simulink model "Flightgear_Tester"  (Simulink 7.8)
settings: Solver=FixedStepDiscrete  SolverMode=SingleTasking  StartTime=0.0  StopTime=inf  FixedStep=dt_sim  RelTol=1e-3
values from neighbouring files (symbols this model uses):
  D = 1    [Init.m]
  dt_sim = 0.005    [Init.m]
undefined symbols (not defined in the file or in its folder): scenario, vis, waitfortreal
settings Model: Creator=ft14sl  LastModifiedBy=ft14sl
settings DataIOCC: LimitDataPoints=off  SaveOutput=off  SignalLogging=off  DSMLogging=off  SaveTime=off
settings DebuggingCC: ConsistencyChecking=error  SignalInfNanChecking=error  SignalRangeChecking=error  AlgebraicLoopMsg=error  ArtificialAlgebraicLoopMsg=error  SaveWithDisabledLinksMsg=error  SaveWithParameterizedLinksMsg=error  UnderspecifiedInitializationDetection=Simplified  MergeDetectMultiDrivingBlocksExec=error  BlockPriorityViolationMsg=error  MinStepSizeMsg=error  TimeAdjustmentMsg=warning  SolverPrmCheckMsg=error  InheritedTsInSrcMsg=error  DiscreteInheritContinuousMsg=error  SingleTaskRateTransMsg=error  TasksWithSamePriorityMsg=error  SigSpecEnsureSampleTimeMsg=error  CheckMatrixSingularityMsg=error  IntegerOverflowMsg=error  ParameterUnderflowMsg=error  ParameterPrecisionLossMsg=error  ParameterTunabilityLossMsg=error  FixptConstUnderflowMsg=error  FixptConstOverflowMsg=error  FixptConstPrecisionLossMsg=error  UnderSpecifiedDataTypeMsg=error  UnnecessaryDatatypeConvMsg=warning  VectorMatrixConversionMsg=error  SignalLabelMismatchMsg=error  UnconnectedInputMsg=error  UnconnectedOutputMsg=error  UnconnectedLineMsg=error  SFcnCompatibilityMsg=error  UniqueDataStoreMsg=error  BusObjectLabelMismatch=error  RootOutportRequireBusObject=error  ModelReferenceIOMsg=error  ModelReferenceVersionMismatchMessage=error  ModelReferenceIOMismatchMessage=error  ModelReferenceCSMismatchMessage=error  UnknownTsInhSupMsg=error  ModelReferenceDataLoggingMessage=error  SimStateInterfaceChecksumMismatchMsg=error  StrictBusMsg=ErrorOnBusTreatedAsVector  NonBusSignalsTreatedAsBus=error  SFUnusedDataAndEventsDiag=error  SFUnexpectedBacktrackingDiag=error  SFInvalidInputDataAccessInChartInitDiag=error  SFNoUnconditionalDefaultTransitionDiag=error  SFTransitionOutsideNaturalParentDiag=error  SFUnconditionalTransitionShadowingDiag=error

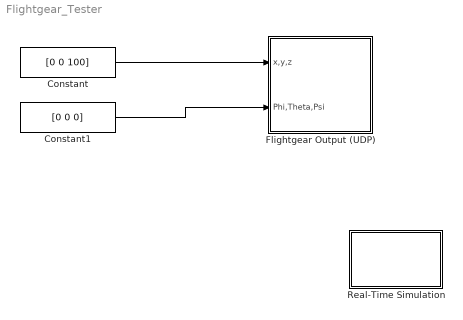
== system Flightgear_Tester ==
  Constant : Constant  Value=[0 0 100]
  Constant1 : Constant  Value=[0 0 0]
  Flightgear Output (UDP) : Subsystem  TreatAsAtomicUnit=on
  Real-Time Simulation : Subsystem
      mask Display: disp('SL RT')
  wires:
  Constant/1 -> Flightgear Output (UDP)/1(x,y,z)
  Constant1/1 -> Flightgear Output (UDP)/2(Phi,Theta,Psi)

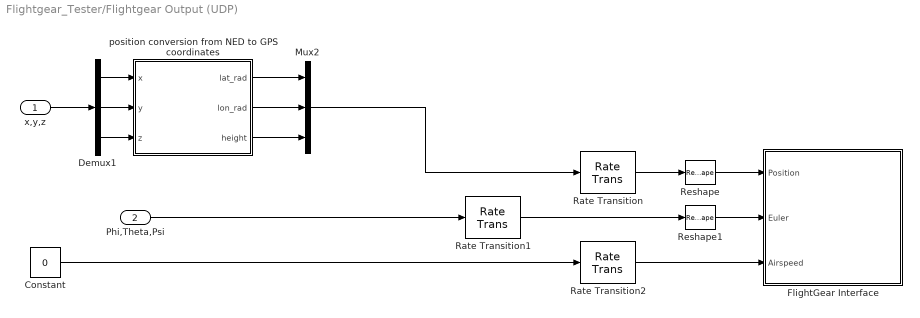
== system Flightgear_Tester/Flightgear Output (UDP) ==
  x,y,z : Inport
  Phi,Theta,Psi : Inport  Port=2
  Constant : Constant  Value=0
  Demux1 : Demux  Outputs=3
  FlightGear Interface : Subsystem  mask(FlightGear interface){hostname=vis.IP_fg, port=vis.PORT_fg, tsamp=vis.dt_vis}
      mask prompts: hostname "Host name:"; tsamp "Sample time:"
      mask help: FlightGear Flight Simulator Interface that provides a visual output of the aircraft position and attitude.
      mask Help:
      | The block provides position and attitude information to FlightGear Flight Simulator for visual output of the aircraft behavior.
      | <P><B>Parameters:</B>
      | <LI>Sample time: the sample time at which data is sent to FlightGear;</LI>
      | <LI>Host name: the name or IP address of the machine on which FlightGear is running.</LI></P>
      | <P><B>Inputs:</B>
      | <LI> the 3x1 vector of geographic position;</LI>
      | <LI> the 3x1 vector of Euler angles;</LI>
      | <LI> scalar number representing airspeed.</LI></P>
  Mux2 : Mux  Inputs=3
  Rate Transition : RateTransition
  Rate Transition1 : RateTransition
  Rate Transition2 : RateTransition
  Reshape : Reshape  OutputDimensionality=Column vector (2-D)
  Reshape1 : Reshape  OutputDimensionality=Column vector (2-D)
  position conversion from NED to GPS coordinates : Subsystem  mask{dRefLat=scenario.dRefLat, dRefLon=scenario.dRefLon, dRefAlt=scenario.dRefAlt, dt_sim=dt_sim}
      mask prompts: dRefLat "Reference Latitude (dRefLat) in rad"; dRefLon "Reference Longitude (dRefLon) in rad"; dRefAlt "Reference altitude (dRefAlt)  in rad"; dt_sim "Sample Time"
      mask init:
      | %WGS-84 semimajor axis_m
      | C_WGS84_a = 6378137.0;
      | %WGS-84 numerical eccentricity
      | C_WGS84_ECC_2=0.006694379992;
      | 
      | %small error
      | sqsinphi = (sin(dRefLat))*(sin(dRefLat)); %Phi, lateral
      | 
      | Rn = C_WGS84_a * ( 1.0 - C_WGS84_ECC_2 ) * (1.0 - C_WGS84_ECC_2*sqsinphi )^(-1.5);
      | Re = C_WGS84_a / sqrt( 1.0 - C_WGS84_ECC_2 * sqsinphi);
  wires:
  Rate Transition1/1 -> Reshape1/1
  Reshape1/1 -> FlightGear Interface/2(Euler)
  Reshape/1 -> FlightGear Interface/1(Position)
  Rate Transition2/1 -> FlightGear Interface/3(Airspeed)
  Rate Transition/1 -> Reshape/1
  Constant/1 -> Rate Transition2/1
  Phi,Theta,Psi/1 -> Rate Transition1/1
  x,y,z/1 -> Demux1/1
  Demux1/1 -> position conversion from NED to GPS coordinates/1(x)
  Demux1/2 -> position conversion from NED to GPS coordinates/2(y)
  Demux1/3 -> position conversion from NED to GPS coordinates/3(z)
  position conversion from NED to GPS coordinates/1(lat_rad) -> Mux2/1
  position conversion from NED to GPS coordinates/2(lon_rad) -> Mux2/2
  position conversion from NED to GPS coordinates/3(height) -> Mux2/3
  Mux2/1 -> Rate Transition/1

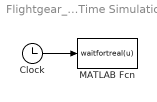
== system Flightgear_Tester/Real-Time Simulation ==
  Clock : Clock
  MATLAB Fcn : MATLABFcn  MATLABFcn=waitfortreal(u)  OutputDimensions=0
  wires:
  Clock/1 -> MATLAB Fcn/1

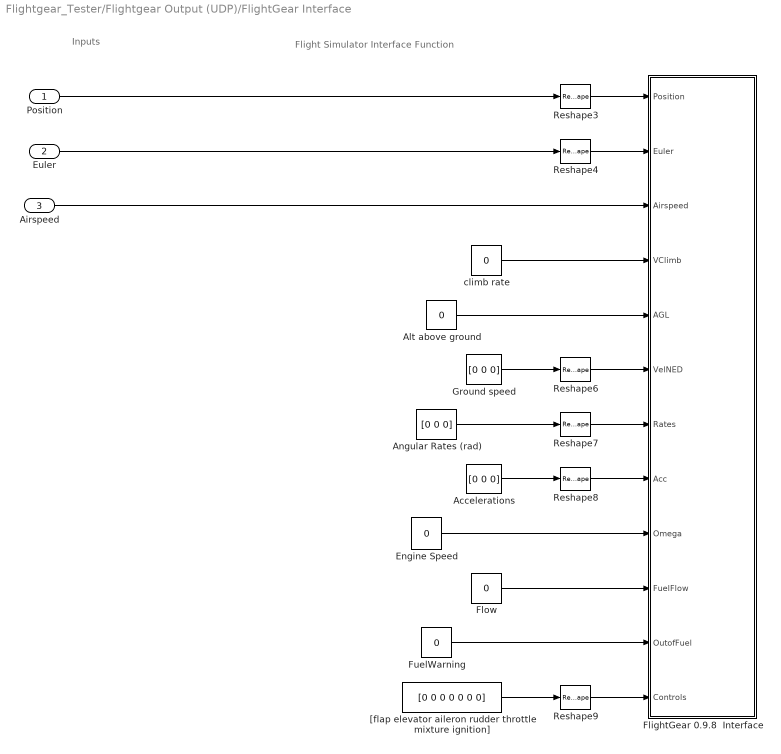
== system Flightgear_Tester/Flightgear Output (UDP)/FlightGear Interface ==
  note: Inputs
  note: Flight Simulator Interface Function
  Position : Inport  OutDataTypeStr=double  PortDimensions=[3 1]
  Euler : Inport  Port=2  OutDataTypeStr=double  PortDimensions=[3 1]
  Airspeed : Inport  Port=3  OutDataTypeStr=double  PortDimensions=1
  Accelerations : Constant  Value=[0 0 0]
  Alt above ground : Constant  Value=0
  Angular Rates (rad) : Constant  Value=[0 0 0]
  Engine Speed : Constant  Value=0
  FlightGear 0.9.8  Interface : Subsystem  mask(FlightGear 0.9.8 interface){hostname=hostname, port=port, tsamp=tsamp}
      mask prompts: hostname "Host name:"; tsamp "Sample time:"
      mask help:
      | FlightGear Flight Simulator Interface that provides a visual output of the aircraft position and attitude.
      | This driver can be used with FlightGear 0.9.8 only.
      mask Help:
      | The block provides position and attitude information to FlightGear Flight Simulator 0.9.8 for visual output of the aircraft behavior.
      | <P><B>Parameters:</B>
      | <LI>Sample time: the sample time at which data is sent to FlightGear;</LI>
      | <LI>Host name: the name or IP address of the machine on which FlightGear is running.</LI>
      | <LI>Port: the port number on the host machine.</LI>
      | </P>
      | <P><B>Inputs:</B>
      | <LI>Position =  the 3x1 vector of geographic position in [rad rad m];</LI>
      | <LI>Euler =  the 3x1 vector of Euler angles in radians;</LI>
      | <LI>Airspeed =  scalar number representing airspeed, in m/s;</LI>
      | <LI>VClimb = the climb rate, in m/s;</LI>
      | <LI>AGL = the altitude above ground, in meters;</LI>
      | <LI>VelNED = the 3x1 vector of groundspeed, in m/s;</LI>
      | <LI>Rates = the 3x1 vector of angular rates, in rad/s;</LI>
      | <LI>Acc = the 3x1 vector of body accelerations, in m/s^2;</LI>
      | <LI>Omega = the engine speed,in rad/s;</LI>
      | <LI>FuelFlow = the instananeous fuel flow, in grams per hour;</LI>
      | <LI>OutofFuel = set it to 1 to disable engine noise in FlightGear, otherwise set it to 0;</LI>
      | <LI>Controls = the 7x1 vector of aircraft controls [flap elevator aileron rudder throttle mixture ignition]; the first 4 aerodynamic controls should be normalized to [-1, 1].</LI>
      | </P>
  Flow : Constant  Value=0
  FuelWarning : Constant  Value=0
  Ground speed : Constant  Value=[0 0 0]
  Reshape{3..4,6..9} (6 alike) : Reshape  OutputDimensionality=Column vector (2-D)
  "[flap elevator aileron rudder throttle mixture ignition]" : Constant  Value=[0 0 0 0 0 0 0]
  climb rate : Constant  Value=0
  wires:
  Reshape9/1 -> FlightGear 0.9.8  Interface/12(Controls)
  Reshape8/1 -> FlightGear 0.9.8  Interface/8(Acc)
  Reshape7/1 -> FlightGear 0.9.8  Interface/7(Rates)
  Reshape6/1 -> FlightGear 0.9.8  Interface/6(VelNED)
  Reshape4/1 -> FlightGear 0.9.8  Interface/2(Euler)
  Reshape3/1 -> FlightGear 0.9.8  Interface/1(Position)
  "[flap elevator aileron rudder throttle mixture ignition]"/1 -> Reshape9/1
  FuelWarning/1 -> FlightGear 0.9.8  Interface/11(OutofFuel)
  Flow/1 -> FlightGear 0.9.8  Interface/10(FuelFlow)
  Engine Speed/1 -> FlightGear 0.9.8  Interface/9(Omega)
  Accelerations/1 -> Reshape8/1
  Angular Rates (rad)/1 -> Reshape7/1
  Ground speed/1 -> Reshape6/1
  Alt above ground/1 -> FlightGear 0.9.8  Interface/5(AGL)
  climb rate/1 -> FlightGear 0.9.8  Interface/4(VClimb)
  Position/1 -> Reshape3/1
  Euler/1 -> Reshape4/1
  Airspeed/1 -> FlightGear 0.9.8  Interface/3(Airspeed)

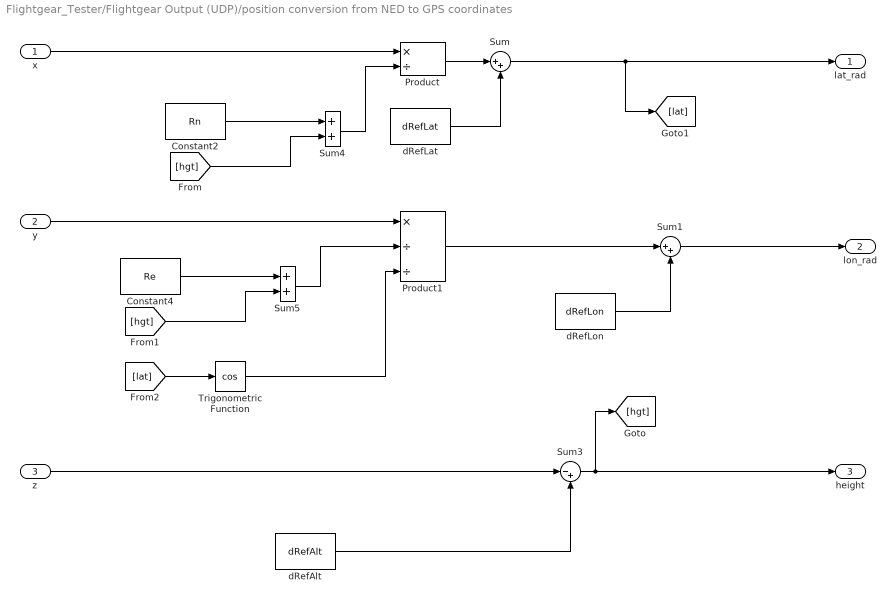
== system Flightgear_Tester/Flightgear Output (UDP)/position conversion from NED to GPS coordinates ==
  x : Inport
  y : Inport  Port=2
  z : Inport  Port=3
  Constant2 : Constant  Value=Rn  SampleTime=dt_sim
  Constant4 : Constant  Value=Re  SampleTime=dt_sim
  Product : Product  Inputs=*/  InputSameDT=on  OutDataTypeStr=Inherit: Same as first input
  Product1 : Product  Inputs=*//  InputSameDT=on  OutDataTypeStr=Inherit: Same as first input
  Sum : Sum  Inputs=|++  SaturateOnIntegerOverflow=on  InputSameDT=on  OutDataTypeStr=Inherit: Same as first input
  Sum1 : Sum  Inputs=|++  SaturateOnIntegerOverflow=on  InputSameDT=on  OutDataTypeStr=Inherit: Same as first input
  Sum3 : Sum  Inputs=|-+  SaturateOnIntegerOverflow=on  InputSameDT=on  OutDataTypeStr=Inherit: Same as first input
  Sum4 : Sum  SaturateOnIntegerOverflow=on  InputSameDT=on  OutDataTypeStr=Inherit: Same as first input
  Sum5 : Sum  SaturateOnIntegerOverflow=on  InputSameDT=on  OutDataTypeStr=Inherit: Same as first input
  Trigonometric Function : Trigonometry  Operator=cos
  dRefAlt : Constant  Value=dRefAlt  SampleTime=dt_sim
  dRefLat : Constant  Value=dRefLat  SampleTime=dt_sim
  dRefLon : Constant  Value=dRefLon  SampleTime=dt_sim
  lat_rad : Outport
  lon_rad : Outport  Port=2
  height : Outport  Port=3
  wires:
  Trigonometric Function/1 -> Product1/3
  [lat] -> Trigonometric Function/1
  [hgt] -> Sum5/2
  dRefLon/1 -> Sum1/2
  Sum5/1 -> Product1/2
  Constant4/1 -> Sum5/1
  Sum1/1 -> lon_rad/1
  Product1/1 -> Sum1/1
  [hgt] -> Sum4/2
  dRefLat/1 -> Sum/2
  Sum4/1 -> Product/2
  Constant2/1 -> Sum4/1
  Sum3/1 -> [hgt], height/1
  dRefAlt/1 -> Sum3/2
  Sum/1 -> [lat], lat_rad/1
  Product/1 -> Sum/1
  x/1 -> Product/1
  y/1 -> Product1/1
  z/1 -> Sum3/1

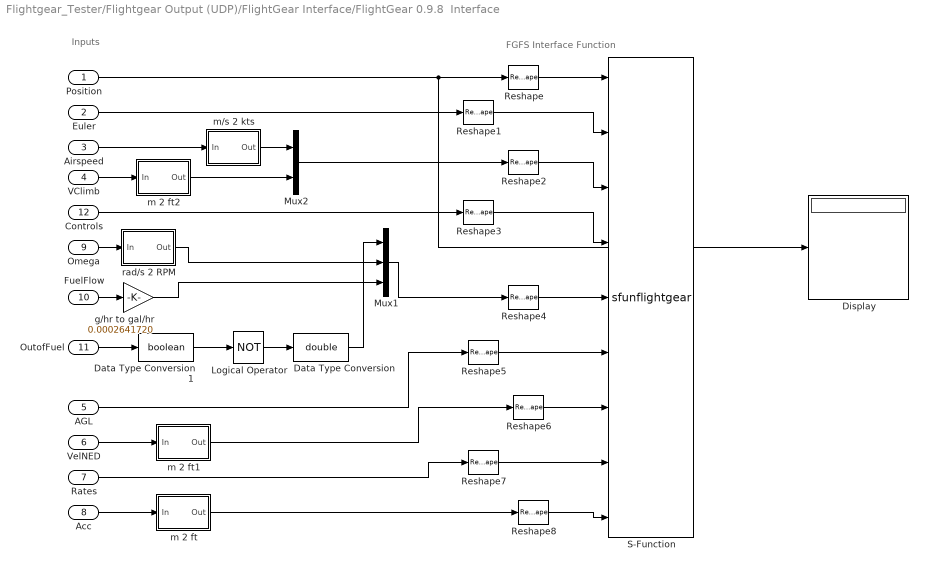
== system Flightgear_Tester/Flightgear Output (UDP)/FlightGear Interface/FlightGear 0.9.8  Interface ==
  note: FGFS Interface Function
  note: Inputs
  Position : Inport  OutDataTypeStr=double  PortDimensions=[3 1]
  Euler : Inport  Port=2  OutDataTypeStr=double  PortDimensions=[3 1]
  Airspeed : Inport  Port=3  OutDataTypeStr=double  PortDimensions=1
  VClimb : Inport  Port=4  OutDataTypeStr=double  PortDimensions=1
  AGL : Inport  Port=5  OutDataTypeStr=double  PortDimensions=1
  VelNED : Inport  Port=6  OutDataTypeStr=double  PortDimensions=[3 1]
  Rates : Inport  Port=7  OutDataTypeStr=double  PortDimensions=[3 1]
  Acc : Inport  Port=8  OutDataTypeStr=double  PortDimensions=[3 1]
  Omega : Inport  Port=9  OutDataTypeStr=double  PortDimensions=1
  FuelFlow : Inport  Port=10  OutDataTypeStr=double  PortDimensions=1
  OutofFuel : Inport  Port=11  OutDataTypeStr=double  PortDimensions=1
  Controls : Inport  Port=12  OutDataTypeStr=double  PortDimensions=[7 1]
  Data Type Conversion : DataTypeConversion  OutDataTypeStr=double  SaturateOnIntegerOverflow=on  RndMeth=Zero
  Data Type Conversion1 : DataTypeConversion  OutDataTypeStr=boolean  SaturateOnIntegerOverflow=on  RndMeth=Zero
  Display : Display
  Logical Operator : Logic  Operator=NOT
  Mux1 : Mux  Inputs=3
  Mux2 : Mux  Inputs=2
  Reshape{,1..8} (9 alike) : Reshape
  S-Function : S-Function  FunctionName=sfunflightgear  Parameters=tsamp,hostname,port  EnableBusSupport=off
  g/hr to gal/hr : Gain  Gain=0.0002641720  SaturateOnIntegerOverflow=on  OutDataTypeStr=Inherit: Same as input  ParamDataTypeStr=Inherit: Same as input
  m 2 ft : Subsystem
      mask Type: Meters to feet
      mask Description: Convert meters to feet.
      mask Help:
      | Meters to feet conversion.
      | <P><B>Input:</B> distance in meters;</P>
      | <P><B>Output:</B> distance in feet.</P>
      mask Display: disp('M       FT');
  m 2 ft1 : Subsystem
      mask Type: Meters to feet
      mask Description: Convert meters to feet.
      mask Help:
      | Meters to feet conversion.
      | <P><B>Input:</B> distance in meters;</P>
      | <P><B>Output:</B> distance in feet.</P>
      mask Display: disp('M       FT');
  m 2 ft2 : Subsystem
      mask Type: Meters to feet
      mask Description: Convert meters to feet.
      mask Help:
      | Meters to feet conversion.
      | <P><B>Input:</B> distance in meters;</P>
      | <P><B>Output:</B> distance in feet.</P>
      mask Display: disp('M       FT');
  m/s 2 kts : Subsystem
      mask Type: Meters per second to knots
      mask Description: Convert meters per second to knots.
      mask Help:
      | Meters per second to knots conversion.
      | <P><B>Input:</B> speed in meters per second;</P>
      | <P><B>Output:</B> speed in knots.</P>
      mask Display: disp('M/S  KTS');
  rad/s 2 RPM : Subsystem
      mask Type: rad/s to RPM
      mask Description: Convert radians-per-second to rotations-per-minute.
      mask Help:
      | Radians per second to rotations per minute conversion.
      | <P><B>Input:</B> angular speed in radians per second;</P>
      | <P><B>Output:</B> angular speed in rotations per minute.</P>
  wires:
  Reshape8/1 -> S-Function/9
  Reshape7/1 -> S-Function/8
  Reshape6/1 -> S-Function/7
  Reshape5/1 -> S-Function/6
  Reshape4/1 -> S-Function/5
  Reshape3/1 -> S-Function/4
  Reshape2/1 -> S-Function/3
  Reshape1/1 -> S-Function/2
  Reshape/1 -> S-Function/1
  Data Type Conversion1/1 -> Logical Operator/1
  VClimb/1 -> m 2 ft2/1(In)
  Airspeed/1 -> m/s 2 kts/1(In)
  Euler/1 -> Reshape1/1
  Position/1 -> Reshape/1, Display/1
  Mux2/1 -> Reshape2/1
  Controls/1 -> Reshape3/1
  Omega/1 -> rad/s 2 RPM/1(In)
  OutofFuel/1 -> Data Type Conversion1/1
  rad/s 2 RPM/1(Out) -> Mux1/2
  FuelFlow/1 -> g/hr to gal/hr/1
  g/hr to gal/hr/1 -> Mux1/3
  Mux1/1 -> Reshape4/1
  Logical Operator/1 -> Data Type Conversion/1
  Data Type Conversion/1 -> Mux1/1
  AGL/1 -> Reshape5/1
  VelNED/1 -> m 2 ft1/1(In)
  Rates/1 -> Reshape7/1
  Acc/1 -> m 2 ft/1(In)
  m 2 ft/1(Out) -> Reshape8/1
  m 2 ft1/1(Out) -> Reshape6/1
  m 2 ft2/1(Out) -> Mux2/2
  m/s 2 kts/1(Out) -> Mux2/1

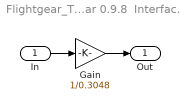
== system Flightgear_Tester/Flightgear Output (UDP)/FlightGear Interface/FlightGear 0.9.8  Interface/m 2 ft ==
  In : Inport
  Gain : Gain  Gain=1/0.3048  SaturateOnIntegerOverflow=on  OutDataTypeStr=Inherit: Same as input  ParamDataTypeStr=Inherit: Same as input
  Out : Outport
  wires:
  Gain/1 -> Out/1
  In/1 -> Gain/1

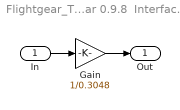
== system Flightgear_Tester/Flightgear Output (UDP)/FlightGear Interface/FlightGear 0.9.8  Interface/m 2 ft1 ==
  In : Inport
  Gain : Gain  Gain=1/0.3048  SaturateOnIntegerOverflow=on  OutDataTypeStr=Inherit: Same as input  ParamDataTypeStr=Inherit: Same as input
  Out : Outport
  wires:
  Gain/1 -> Out/1
  In/1 -> Gain/1

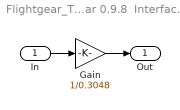
== system Flightgear_Tester/Flightgear Output (UDP)/FlightGear Interface/FlightGear 0.9.8  Interface/m 2 ft2 ==
  In : Inport
  Gain : Gain  Gain=1/0.3048  SaturateOnIntegerOverflow=on  OutDataTypeStr=Inherit: Same as input  ParamDataTypeStr=Inherit: Same as input
  Out : Outport
  wires:
  Gain/1 -> Out/1
  In/1 -> Gain/1

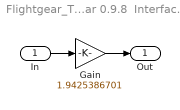
== system Flightgear_Tester/Flightgear Output (UDP)/FlightGear Interface/FlightGear 0.9.8  Interface/m/s 2 kts ==
  In : Inport
  Gain : Gain  Gain=1.9425386701  SaturateOnIntegerOverflow=on  OutDataTypeStr=Inherit: Same as input  ParamDataTypeStr=Inherit: Same as input
  Out : Outport
  wires:
  In/1 -> Gain/1
  Gain/1 -> Out/1

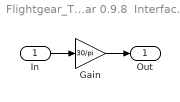
== system Flightgear_Tester/Flightgear Output (UDP)/FlightGear Interface/FlightGear 0.9.8  Interface/rad/s 2 RPM ==
  In : Inport
  Gain : Gain  Gain=30/pi  SaturateOnIntegerOverflow=on  OutDataTypeStr=Inherit: Same as input  ParamDataTypeStr=Inherit: Same as input
  Out : Outport
  wires:
  Gain/1 -> Out/1
  In/1 -> Gain/1
